simulink subsystem "Piero_Clase_Model"  (R2023b)
settings: Solver=VariableStepAuto  StartTime=0.0  StopTime=10.0  RelTol=1e-3
settings Model: Creator=javie  LastModifiedBy=javie

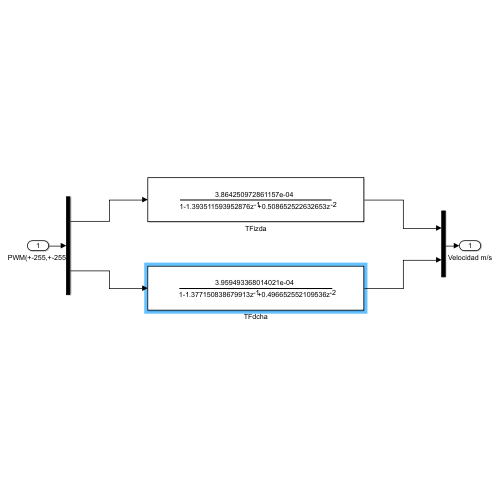
[thumbnail: Simulink's stored preview of the top-level diagram]
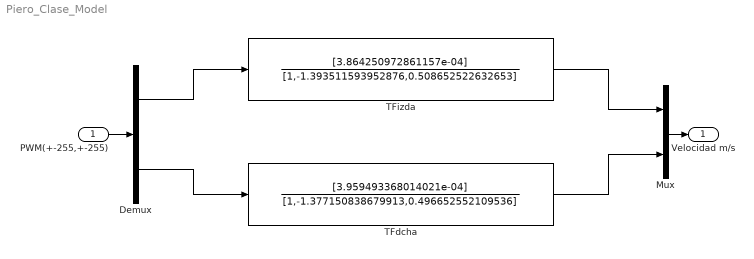
== system Piero_Clase_Model ==
  PWM(+-255,+-255) : Inport
  Demux : Demux  Outputs=2
  Mux : Mux  Inputs=2
  TFdcha : DiscreteFilter  Numerator=[3.959493368014021e-04]  Denominator=[1,-1.377150838679913,0.496652552109536]
  TFizda : DiscreteFilter  Numerator=[3.864250972861157e-04]  Denominator=[1,-1.393511593952876,0.508652522632653]
  Velocidad m/s : Outport
  wires:
  PWM(+-255,+-255)/1 -> Demux/1
  Mux/1 -> Velocidad m/s/1
  Demux/1 -> TFizda/1
  Demux/2 -> TFdcha/1
  TFizda/1 -> Mux/1
  TFdcha/1 -> Mux/2
